simulink model "mct_ut"  (Simulink 8.1)
settings: Solver=FixedStepDiscrete  StartTime=0.0  StopTime=Inf  FixedStep=0.005  RelTol=1e-3
libraries: siltestlib x41, mct x1
settings Model: Creator=xsellart  LastModifiedBy=AT015555
settings DataIOCC: SignalLoggingSaveFormat=Dataset
settings OptimizationCC: ExpressionDepthLimit=128
settings DebuggingCC: FcnCallInpInsideContextMsg=EnableAllAsError
settings GRTTargetCC: CombineOutputUpdateFcns=on  GRTInterface=off

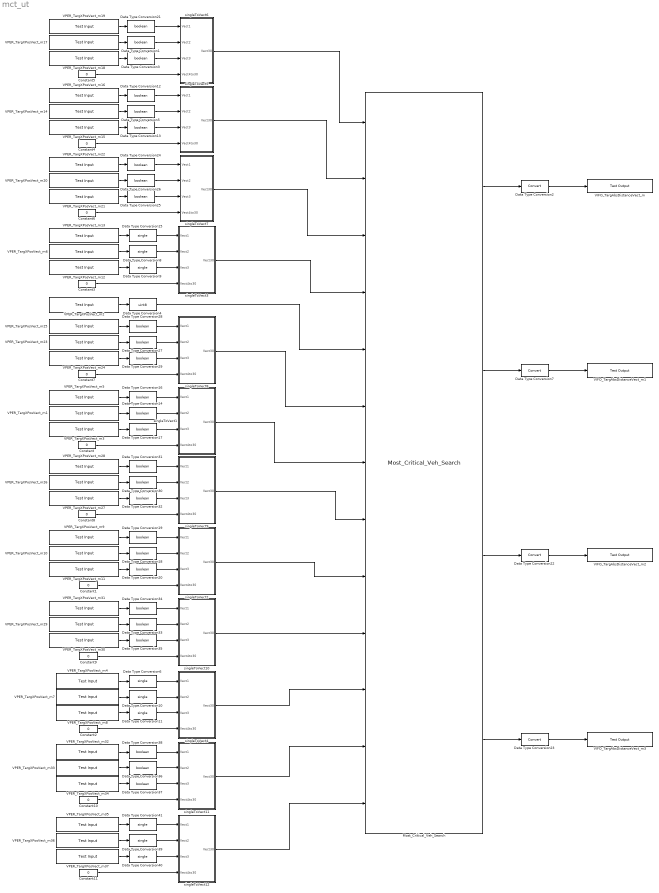
== system mct_ut ==
  Constant{,1,4..10} (9 alike) : Constant  Value=0  OutDataTypeStr=boolean
  Constant11 : Constant  Value=0  OutDataTypeStr=single
  Constant2 : Constant  Value=0  OutDataTypeStr=single
  Constant3 : Constant  Value=0  OutDataTypeStr=single
  Data Type Conversion{1,3,5,12..14,16..21,24..38} (27 alike) : DataTypeConversion  OutDataTypeStr=boolean
  Data Type Conversion{6,8..11,15,39..41} (9 alike) : DataTypeConversion  OutDataTypeStr=single
  Data Type Conversion{2,7,22..23} (4 alike) : DataTypeConversion
  Data Type Conversion4 : DataTypeConversion  OutDataTypeStr=uint8
  Most_Critical_Veh_Search : mct/Most_Critical_Veh_Search
  VIFO_TargAbsDistanceVect_m : siltestlib/Test Output  varname=VIFO_FCWMCTTargId_num  sampletime=-1
  VIFO_TargAbsDistanceVect_m1 : siltestlib/Test Output  varname=VIFO_AEBMCTTargId_num  sampletime=-1
  VIFO_TargAbsDistanceVect_m2 : siltestlib/Test Output  varname=VIFO_ACCMCTTargId_num  sampletime=-1
  VIFO_TargAbsDistanceVect_m3 : siltestlib/Test Output  varname=VIFO_VRUMCTTargId_num  sampletime=-1
  VPER_TargXPosVect_m1 : siltestlib/Test Input  varname=VIFO_ACCTargetIsVehVect30_flg2  sampletime=0.005
  VPER_TargXPosVect_m10 : siltestlib/Test Input  varname=VIFO_AEBTargetSameDirVect30_flg2  sampletime=0.005
  VPER_TargXPosVect_m11 : siltestlib/Test Input  varname=VIFO_AEBTargetSameDirVect30_flg3  sampletime=0.005
  VPER_TargXPosVect_m12 : siltestlib/Test Input  varname=VIFO_TargAbsDistanceVect30_m3  sampletime=0.005
  VPER_TargXPosVect_m13 : siltestlib/Test Input  varname=VIFO_TargAbsDistanceVect30_m1  sampletime=0.005
  VPER_TargXPosVect_m14 : siltestlib/Test Input  varname=VIFO_AEBVehInPathVect30_flg2  sampletime=0.005
  VPER_TargXPosVect_m15 : siltestlib/Test Input  varname=VIFO_AEBVehInPathVect30_flg3  sampletime=0.005
  VPER_TargXPosVect_m16 : siltestlib/Test Input  varname=VIFO_AEBVehInPathVect30_flg1  sampletime=0.005
  VPER_TargXPosVect_m17 : siltestlib/Test Input  varname=VIFO_FCWVehInPathVect30_flg2  sampletime=0.005
  VPER_TargXPosVect_m18 : siltestlib/Test Input  varname=VIFO_FCWVehInPathVect30_flg3  sampletime=0.005
  VPER_TargXPosVect_m19 : siltestlib/Test Input  varname=VIFO_FCWVehInPathVect30_flg1  sampletime=0.005
  VPER_TargXPosVect_m2 : siltestlib/Test Input  varname=VPER_NumberOfTargets_enum  sampletime=0.005
  VPER_TargXPosVect_m20 : siltestlib/Test Input  varname=VIFO_ACCVehInPathVect30_flg2  sampletime=0.005
  VPER_TargXPosVect_m21 : siltestlib/Test Input  varname=VIFO_ACCVehInPathVect30_flg3  sampletime=0.005
  VPER_TargXPosVect_m22 : siltestlib/Test Input  varname=VIFO_ACCVehInPathVect30_flg1  sampletime=0.005
  VPER_TargXPosVect_m23 : siltestlib/Test Input  varname=VIFO_AEBTargetIsVehVect30_flg2  sampletime=0.005
  VPER_TargXPosVect_m24 : siltestlib/Test Input  varname=VIFO_AEBTargetIsVehVect30_flg3  sampletime=0.005
  VPER_TargXPosVect_m25 : siltestlib/Test Input  varname=VIFO_AEBTargetIsVehVect30_flg1  sampletime=0.005
  VPER_TargXPosVect_m26 : siltestlib/Test Input  varname=VIFO_VRUTargetIsPedVect30_flg2  sampletime=0.005
  VPER_TargXPosVect_m27 : siltestlib/Test Input  varname=VIFO_VRUTargetIsPedVect30_flg3  sampletime=0.005
  VPER_TargXPosVect_m28 : siltestlib/Test Input  varname=VIFO_VRUTargetIsPedVect30_flg1  sampletime=0.005
  VPER_TargXPosVect_m29 : siltestlib/Test Input  varname=VIFO_ACCTargetSameDirVect30_flg2  sampletime=0.005
  VPER_TargXPosVect_m3 : siltestlib/Test Input  varname=VIFO_ACCTargetIsVehVect30_flg3  sampletime=0.005
  VPER_TargXPosVect_m30 : siltestlib/Test Input  varname=VIFO_ACCTargetSameDirVect30_flg3  sampletime=0.005
  VPER_TargXPosVect_m31 : siltestlib/Test Input  varname=VIFO_ACCTargetSameDirVect30_flg1  sampletime=0.005
  VPER_TargXPosVect_m32 : siltestlib/Test Input  varname=VIFO_VRUIsPotentialVect30_flg1  sampletime=0.005
  VPER_TargXPosVect_m33 : siltestlib/Test Input  varname=VIFO_VRUIsPotentialVect30_flg2  sampletime=0.005
  VPER_TargXPosVect_m34 : siltestlib/Test Input  varname=VIFO_VRUIsPotentialVect30_flg3  sampletime=0.005
  VPER_TargXPosVect_m35 : siltestlib/Test Input  varname=VIFO_VRUSingleTTCVect30_s1  sampletime=0.005
  VPER_TargXPosVect_m36 : siltestlib/Test Input  varname=VIFO_VRUSingleTTCVect30_s2  sampletime=0.005
  VPER_TargXPosVect_m37 : siltestlib/Test Input  varname=VIFO_VRUSingleTTCVect30_s3  sampletime=0.005
  VPER_TargXPosVect_m4 : siltestlib/Test Input  varname=VPER_TargExisProbVect30_num1  sampletime=0.005
  VPER_TargXPosVect_m5 : siltestlib/Test Input  varname=VIFO_ACCTargetIsVehVect30_flg1  sampletime=0.005
  VPER_TargXPosVect_m6 : siltestlib/Test Input  varname=VIFO_TargAbsDistanceVect30_m2  sampletime=0.005
  VPER_TargXPosVect_m7 : siltestlib/Test Input  varname=VPER_TargExisProbVect30_num2  sampletime=0.005
  VPER_TargXPosVect_m8 : siltestlib/Test Input  varname=VPER_TargExisProbVect30_num3  sampletime=0.005
  VPER_TargXPosVect_m9 : siltestlib/Test Input  varname=VIFO_AEBTargetSameDirVect30_flg1  sampletime=0.005
  singleToVect1 : Subsystem
  singleToVect10 : Subsystem
  singleToVect11 : Subsystem
  singleToVect12 : Subsystem
  singleToVect2 : Subsystem
  singleToVect3 : Subsystem
  singleToVect4 : Subsystem
  singleToVect5 : Subsystem
  singleToVect6 : Subsystem
  singleToVect7 : Subsystem
  singleToVect8 : Subsystem
  singleToVect9 : Subsystem
  wires:
  Most_Critical_Veh_Search/1 -> Data Type Conversion2/1
  Data Type Conversion2/1 -> VIFO_TargAbsDistanceVect_m/1
  VPER_TargXPosVect_m2/1 -> Data Type Conversion4/1
  VPER_TargXPosVect_m4/1 -> Data Type Conversion6/1
  Data Type Conversion6/1 -> singleToVect4/1(Vect1)
  Most_Critical_Veh_Search/2 -> Data Type Conversion7/1
  Data Type Conversion7/1 -> VIFO_TargAbsDistanceVect_m1/1
  VPER_TargXPosVect_m7/1 -> Data Type Conversion10/1
  Data Type Conversion10/1 -> singleToVect4/2(Vect2)
  VPER_TargXPosVect_m8/1 -> Data Type Conversion11/1
  Data Type Conversion11/1 -> singleToVect4/3(Vect3)
  VPER_TargXPosVect_m9/1 -> Data Type Conversion19/1
  Data Type Conversion19/1 -> singleToVect2/1(Vect1)
  VPER_TargXPosVect_m10/1 -> Data Type Conversion18/1
  Data Type Conversion18/1 -> singleToVect2/2(Vect2)
  VPER_TargXPosVect_m11/1 -> Data Type Conversion20/1
  Data Type Conversion20/1 -> singleToVect2/3(Vect3)
  VPER_TargXPosVect_m5/1 -> Data Type Conversion16/1
  Data Type Conversion16/1 -> singleToVect1/1(Vect1)
  VPER_TargXPosVect_m1/1 -> Data Type Conversion14/1
  Data Type Conversion14/1 -> singleToVect1/2(Vect2)
  VPER_TargXPosVect_m3/1 -> Data Type Conversion17/1
  Data Type Conversion17/1 -> singleToVect1/3(Vect3)
  VPER_TargXPosVect_m13/1 -> Data Type Conversion15/1
  Data Type Conversion15/1 -> singleToVect3/1(Vect1)
  VPER_TargXPosVect_m6/1 -> Data Type Conversion8/1
  Data Type Conversion8/1 -> singleToVect3/2(Vect2)
  VPER_TargXPosVect_m12/1 -> Data Type Conversion9/1
  Data Type Conversion9/1 -> singleToVect3/3(Vect3)
  VPER_TargXPosVect_m16/1 -> Data Type Conversion12/1
  Data Type Conversion12/1 -> singleToVect5/1(Vect1)
  VPER_TargXPosVect_m14/1 -> Data Type Conversion5/1
  Data Type Conversion5/1 -> singleToVect5/2(Vect2)
  VPER_TargXPosVect_m15/1 -> Data Type Conversion13/1
  Data Type Conversion13/1 -> singleToVect5/3(Vect3)
  singleToVect5/1(Vect30) -> Most_Critical_Veh_Search/2
  VPER_TargXPosVect_m19/1 -> Data Type Conversion21/1
  Data Type Conversion21/1 -> singleToVect6/1(Vect1)
  VPER_TargXPosVect_m17/1 -> Data Type Conversion1/1
  Data Type Conversion1/1 -> singleToVect6/2(Vect2)
  VPER_TargXPosVect_m18/1 -> Data Type Conversion3/1
  Data Type Conversion3/1 -> singleToVect6/3(Vect3)
  singleToVect6/1(Vect30) -> Most_Critical_Veh_Search/1
  Constant/1 -> singleToVect1/4(Vect4to30)
  Constant1/1 -> singleToVect2/4(Vect4to30)
  Constant2/1 -> singleToVect4/4(Vect4to30)
  Constant3/1 -> singleToVect3/4(Vect4to30)
  Constant4/1 -> singleToVect5/4(Vect4to30)
  Constant5/1 -> singleToVect6/4(Vect4to30)
  Data Type Conversion22/1 -> VIFO_TargAbsDistanceVect_m2/1
  Data Type Conversion23/1 -> VIFO_TargAbsDistanceVect_m3/1
  Most_Critical_Veh_Search/3 -> Data Type Conversion22/1
  Most_Critical_Veh_Search/4 -> Data Type Conversion23/1
  VPER_TargXPosVect_m22/1 -> Data Type Conversion24/1
  Data Type Conversion24/1 -> singleToVect7/1(Vect1)
  VPER_TargXPosVect_m20/1 -> Data Type Conversion26/1
  Data Type Conversion26/1 -> singleToVect7/2(Vect2)
  VPER_TargXPosVect_m21/1 -> Data Type Conversion25/1
  Data Type Conversion25/1 -> singleToVect7/3(Vect3)
  Constant6/1 -> singleToVect7/4(Vect4to30)
  singleToVect7/1(Vect30) -> Most_Critical_Veh_Search/3
  singleToVect3/1(Vect30) -> Most_Critical_Veh_Search/4
  Data Type Conversion4/1 -> Most_Critical_Veh_Search/5
  VPER_TargXPosVect_m25/1 -> Data Type Conversion28/1
  Data Type Conversion28/1 -> singleToVect8/1(Vect1)
  VPER_TargXPosVect_m23/1 -> Data Type Conversion27/1
  Data Type Conversion27/1 -> singleToVect8/2(Vect2)
  VPER_TargXPosVect_m24/1 -> Data Type Conversion29/1
  Data Type Conversion29/1 -> singleToVect8/3(Vect3)
  Constant7/1 -> singleToVect8/4(Vect4to30)
  singleToVect8/1(Vect30) -> Most_Critical_Veh_Search/6
  singleToVect1/1(Vect30) -> Most_Critical_Veh_Search/7
  VPER_TargXPosVect_m28/1 -> Data Type Conversion31/1
  Data Type Conversion31/1 -> singleToVect9/1(Vect1)
  VPER_TargXPosVect_m26/1 -> Data Type Conversion30/1
  Data Type Conversion30/1 -> singleToVect9/2(Vect2)
  VPER_TargXPosVect_m27/1 -> Data Type Conversion32/1
  Data Type Conversion32/1 -> singleToVect9/3(Vect3)
  Constant8/1 -> singleToVect9/4(Vect4to30)
  singleToVect9/1(Vect30) -> Most_Critical_Veh_Search/8
  singleToVect2/1(Vect30) -> Most_Critical_Veh_Search/9
  VPER_TargXPosVect_m31/1 -> Data Type Conversion34/1
  Data Type Conversion34/1 -> singleToVect10/1(Vect1)
  VPER_TargXPosVect_m29/1 -> Data Type Conversion33/1
  Data Type Conversion33/1 -> singleToVect10/2(Vect2)
  VPER_TargXPosVect_m30/1 -> Data Type Conversion35/1
  Data Type Conversion35/1 -> singleToVect10/3(Vect3)
  Constant9/1 -> singleToVect10/4(Vect4to30)
  singleToVect10/1(Vect30) -> Most_Critical_Veh_Search/10
  VPER_TargXPosVect_m32/1 -> Data Type Conversion38/1
  Data Type Conversion38/1 -> singleToVect11/1(Vect1)
  VPER_TargXPosVect_m33/1 -> Data Type Conversion36/1
  Data Type Conversion36/1 -> singleToVect11/2(Vect2)
  VPER_TargXPosVect_m34/1 -> Data Type Conversion37/1
  Data Type Conversion37/1 -> singleToVect11/3(Vect3)
  Constant10/1 -> singleToVect11/4(Vect4to30)
  VPER_TargXPosVect_m35/1 -> Data Type Conversion41/1
  Data Type Conversion41/1 -> singleToVect12/1(Vect1)
  VPER_TargXPosVect_m36/1 -> Data Type Conversion39/1
  Data Type Conversion39/1 -> singleToVect12/2(Vect2)
  VPER_TargXPosVect_m37/1 -> Data Type Conversion40/1
  Data Type Conversion40/1 -> singleToVect12/3(Vect3)
  Constant11/1 -> singleToVect12/4(Vect4to30)
  singleToVect12/1(Vect30) -> Most_Critical_Veh_Search/13
  singleToVect4/1(Vect30) -> Most_Critical_Veh_Search/11
  singleToVect11/1(Vect30) -> Most_Critical_Veh_Search/12

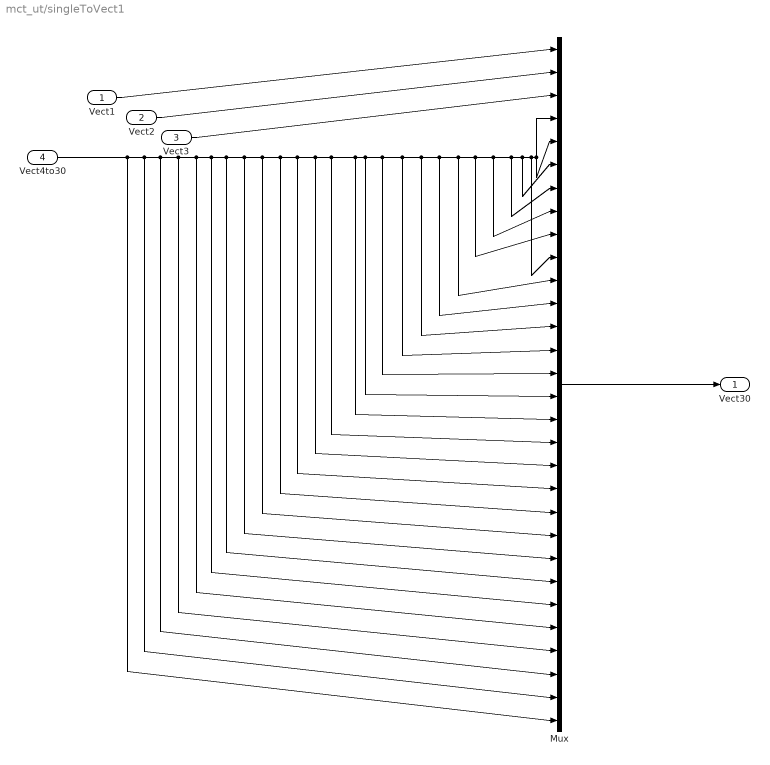
== system mct_ut/singleToVect1 ==
  Vect1 : Inport
  Vect2 : Inport  Port=2
  Vect3 : Inport  Port=3
  Vect4to30 : Inport  Port=4
  Mux : Mux  Inputs=30
  Vect30 : Outport
  wires:
  Mux/1 -> Vect30/1
  Vect4to30/1 -> Mux/30, Mux/29, Mux/28, Mux/27, Mux/26, Mux/25, Mux/24, Mux/23, Mux/22, Mux/21, Mux/20, Mux/19, Mux/18, Mux/17, Mux/16, Mux/15, Mux/14, Mux/13, Mux/12, Mux/11, Mux/10, Mux/4, Mux/5, Mux/6, Mux/7, Mux/8, Mux/9
  Vect3/1 -> Mux/3
  Vect2/1 -> Mux/2
  Vect1/1 -> Mux/1

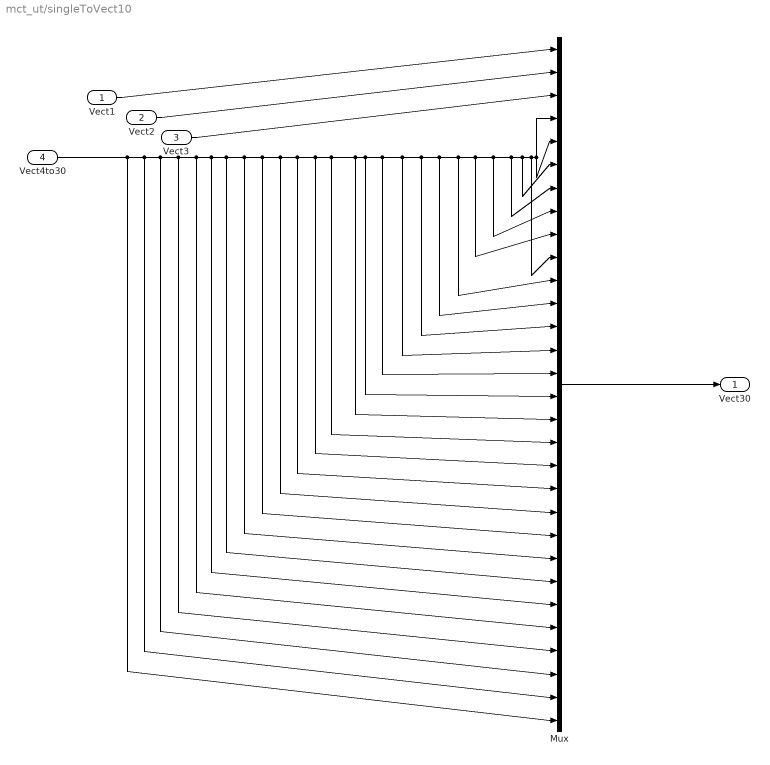
== system mct_ut/singleToVect10 ==
  Vect1 : Inport
  Vect2 : Inport  Port=2
  Vect3 : Inport  Port=3
  Vect4to30 : Inport  Port=4
  Mux : Mux  Inputs=30
  Vect30 : Outport
  wires:
  Vect1/1 -> Mux/1
  Vect2/1 -> Mux/2
  Vect3/1 -> Mux/3
  Vect4to30/1 -> Mux/9, Mux/8, Mux/7, Mux/6, Mux/5, Mux/4, Mux/10, Mux/11, Mux/12, Mux/13, Mux/14, Mux/15, Mux/16, Mux/17, Mux/18, Mux/19, Mux/20, Mux/21, Mux/22, Mux/23, Mux/24, Mux/25, Mux/26, Mux/27, Mux/28, Mux/29, Mux/30
  Mux/1 -> Vect30/1

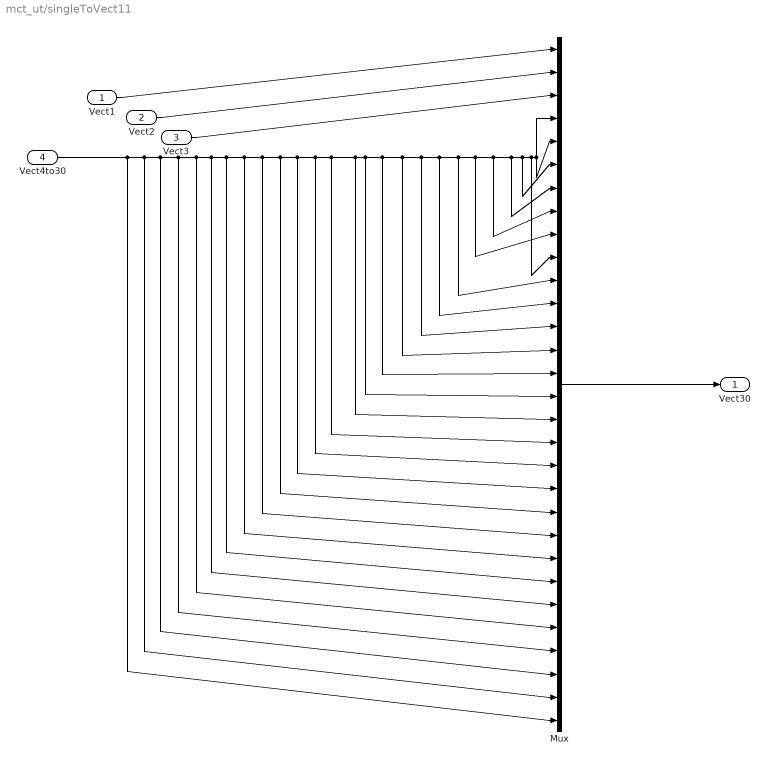
== system mct_ut/singleToVect11 ==
  Vect1 : Inport
  Vect2 : Inport  Port=2
  Vect3 : Inport  Port=3
  Vect4to30 : Inport  Port=4
  Mux : Mux  Inputs=30
  Vect30 : Outport
  wires:
  Vect1/1 -> Mux/1
  Vect2/1 -> Mux/2
  Vect3/1 -> Mux/3
  Vect4to30/1 -> Mux/9, Mux/8, Mux/7, Mux/6, Mux/5, Mux/4, Mux/10, Mux/11, Mux/12, Mux/13, Mux/14, Mux/15, Mux/16, Mux/17, Mux/18, Mux/19, Mux/20, Mux/21, Mux/22, Mux/23, Mux/24, Mux/25, Mux/26, Mux/27, Mux/28, Mux/29, Mux/30
  Mux/1 -> Vect30/1

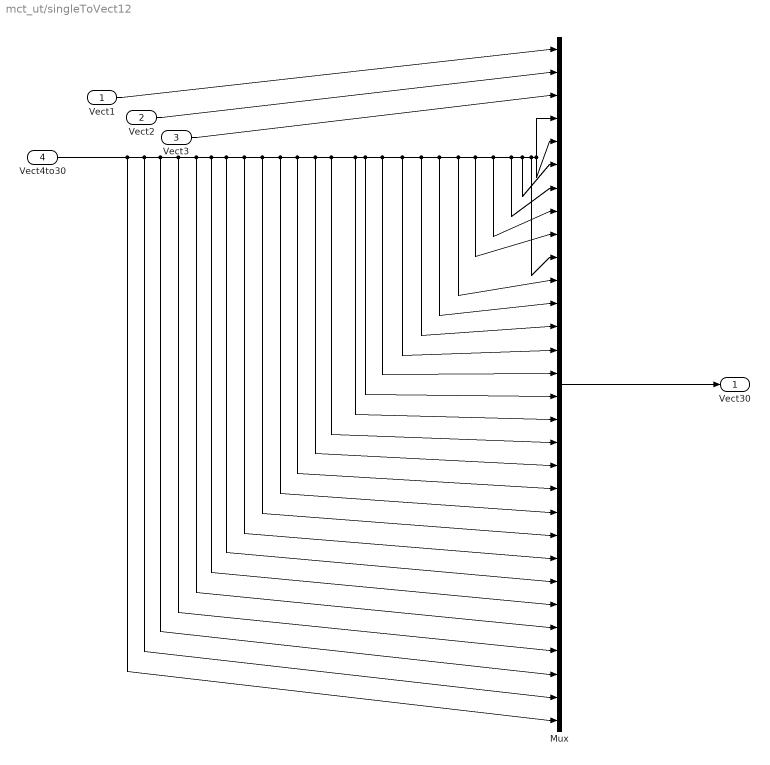
== system mct_ut/singleToVect12 ==
  Vect1 : Inport
  Vect2 : Inport  Port=2
  Vect3 : Inport  Port=3
  Vect4to30 : Inport  Port=4
  Mux : Mux  Inputs=30
  Vect30 : Outport
  wires:
  Mux/1 -> Vect30/1
  Vect4to30/1 -> Mux/30, Mux/29, Mux/28, Mux/27, Mux/26, Mux/25, Mux/24, Mux/23, Mux/22, Mux/21, Mux/20, Mux/19, Mux/18, Mux/17, Mux/16, Mux/15, Mux/14, Mux/13, Mux/12, Mux/11, Mux/10, Mux/4, Mux/5, Mux/6, Mux/7, Mux/8, Mux/9
  Vect3/1 -> Mux/3
  Vect2/1 -> Mux/2
  Vect1/1 -> Mux/1

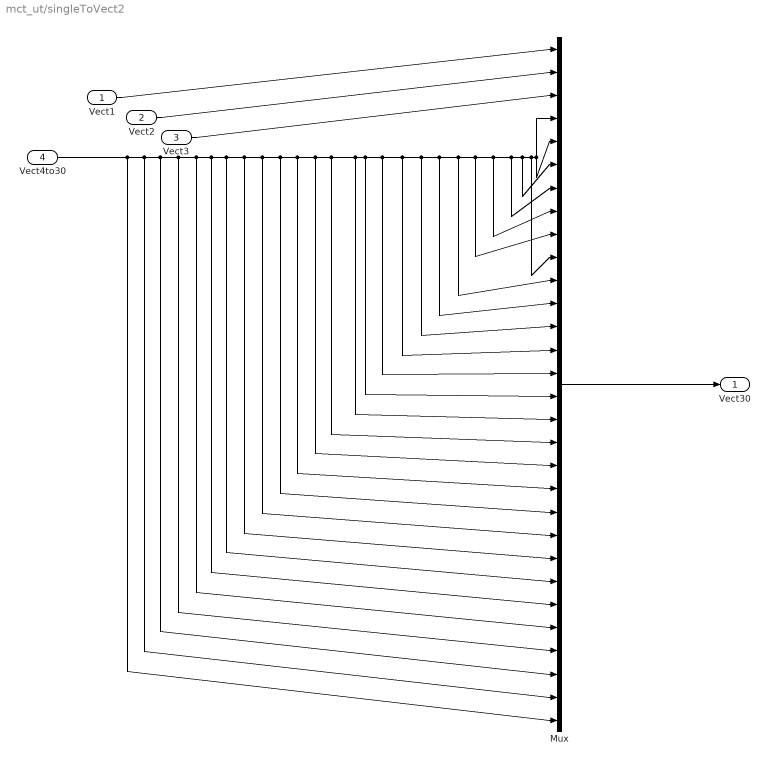
== system mct_ut/singleToVect2 ==
  Vect1 : Inport
  Vect2 : Inport  Port=2
  Vect3 : Inport  Port=3
  Vect4to30 : Inport  Port=4
  Mux : Mux  Inputs=30
  Vect30 : Outport
  wires:
  Mux/1 -> Vect30/1
  Vect4to30/1 -> Mux/30, Mux/29, Mux/28, Mux/27, Mux/26, Mux/25, Mux/24, Mux/23, Mux/22, Mux/21, Mux/20, Mux/19, Mux/18, Mux/17, Mux/16, Mux/15, Mux/14, Mux/13, Mux/12, Mux/11, Mux/10, Mux/4, Mux/5, Mux/6, Mux/7, Mux/8, Mux/9
  Vect3/1 -> Mux/3
  Vect2/1 -> Mux/2
  Vect1/1 -> Mux/1

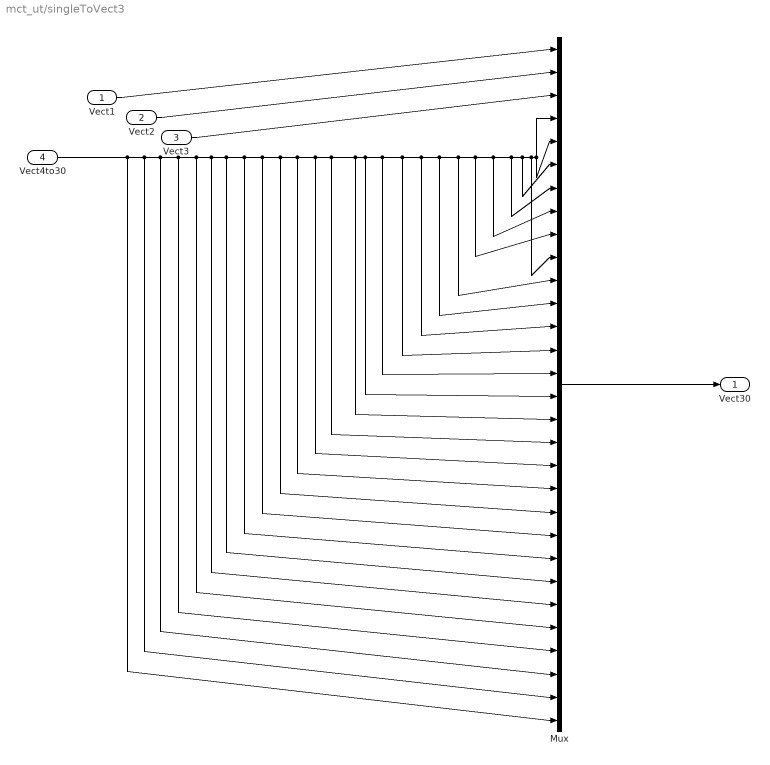
== system mct_ut/singleToVect3 ==
  Vect1 : Inport
  Vect2 : Inport  Port=2
  Vect3 : Inport  Port=3
  Vect4to30 : Inport  Port=4
  Mux : Mux  Inputs=30
  Vect30 : Outport
  wires:
  Mux/1 -> Vect30/1
  Vect4to30/1 -> Mux/30, Mux/29, Mux/28, Mux/27, Mux/26, Mux/25, Mux/24, Mux/23, Mux/22, Mux/21, Mux/20, Mux/19, Mux/18, Mux/17, Mux/16, Mux/15, Mux/14, Mux/13, Mux/12, Mux/11, Mux/10, Mux/4, Mux/5, Mux/6, Mux/7, Mux/8, Mux/9
  Vect3/1 -> Mux/3
  Vect2/1 -> Mux/2
  Vect1/1 -> Mux/1

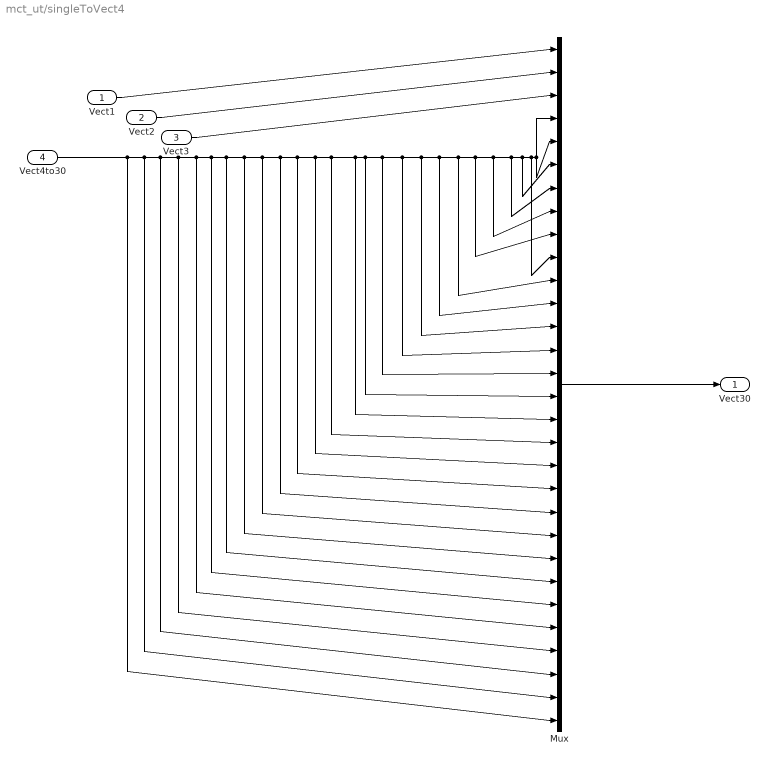
== system mct_ut/singleToVect4 ==
  Vect1 : Inport
  Vect2 : Inport  Port=2
  Vect3 : Inport  Port=3
  Vect4to30 : Inport  Port=4
  Mux : Mux  Inputs=30
  Vect30 : Outport
  wires:
  Mux/1 -> Vect30/1
  Vect4to30/1 -> Mux/30, Mux/29, Mux/28, Mux/27, Mux/26, Mux/25, Mux/24, Mux/23, Mux/22, Mux/21, Mux/20, Mux/19, Mux/18, Mux/17, Mux/16, Mux/15, Mux/14, Mux/13, Mux/12, Mux/11, Mux/10, Mux/4, Mux/5, Mux/6, Mux/7, Mux/8, Mux/9
  Vect3/1 -> Mux/3
  Vect2/1 -> Mux/2
  Vect1/1 -> Mux/1

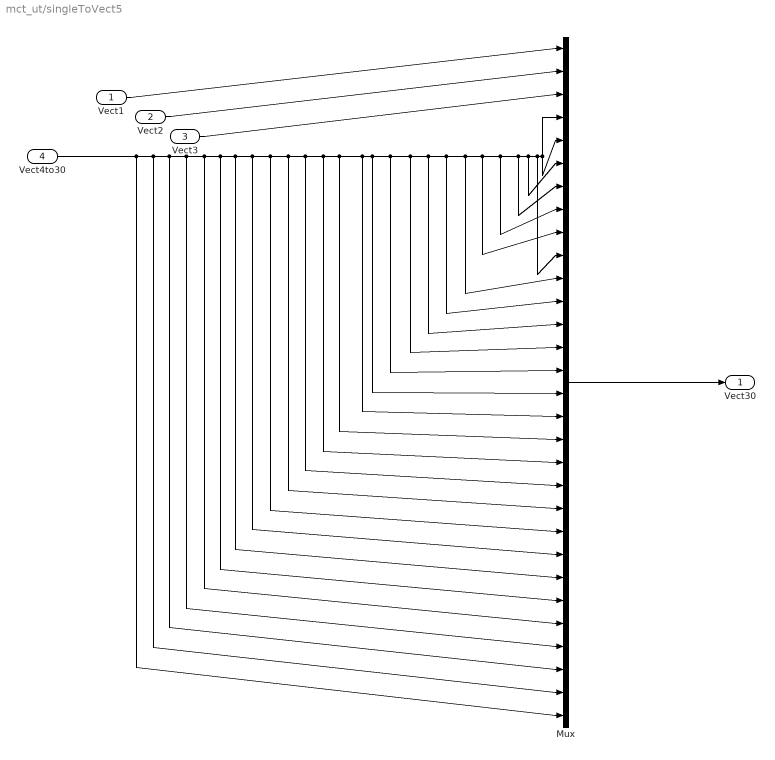
== system mct_ut/singleToVect5 ==
  Vect1 : Inport
  Vect2 : Inport  Port=2
  Vect3 : Inport  Port=3
  Vect4to30 : Inport  Port=4
  Mux : Mux  Inputs=30
  Vect30 : Outport
  wires:
  Mux/1 -> Vect30/1
  Vect4to30/1 -> Mux/30, Mux/29, Mux/28, Mux/27, Mux/26, Mux/25, Mux/24, Mux/23, Mux/22, Mux/21, Mux/20, Mux/19, Mux/18, Mux/17, Mux/16, Mux/15, Mux/14, Mux/13, Mux/12, Mux/11, Mux/10, Mux/4, Mux/5, Mux/6, Mux/7, Mux/8, Mux/9
  Vect3/1 -> Mux/3
  Vect2/1 -> Mux/2
  Vect1/1 -> Mux/1

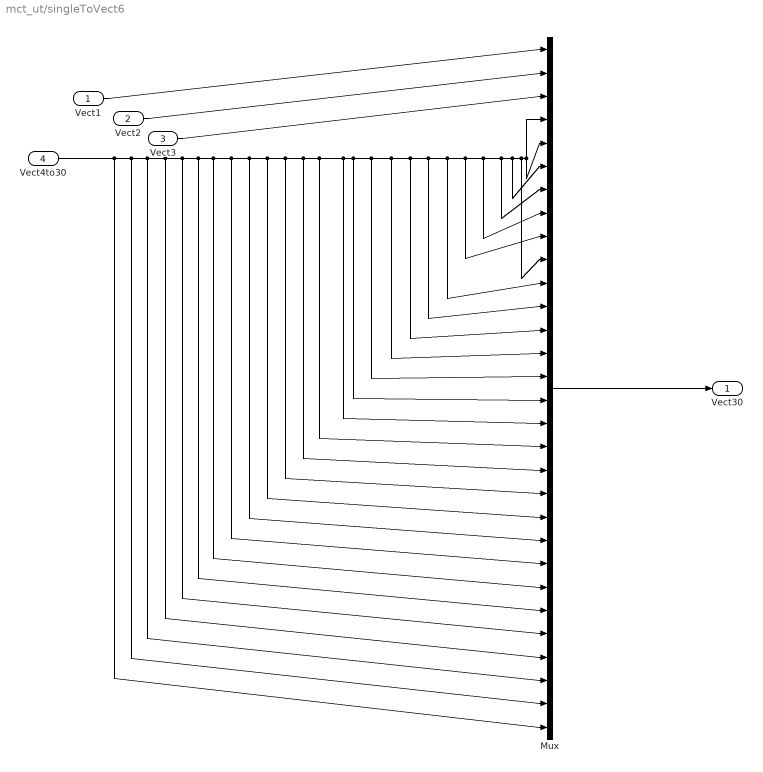
== system mct_ut/singleToVect6 ==
  Vect1 : Inport
  Vect2 : Inport  Port=2
  Vect3 : Inport  Port=3
  Vect4to30 : Inport  Port=4
  Mux : Mux  Inputs=30
  Vect30 : Outport
  wires:
  Mux/1 -> Vect30/1
  Vect4to30/1 -> Mux/30, Mux/29, Mux/28, Mux/27, Mux/26, Mux/25, Mux/24, Mux/23, Mux/22, Mux/21, Mux/20, Mux/19, Mux/18, Mux/17, Mux/16, Mux/15, Mux/14, Mux/13, Mux/12, Mux/11, Mux/10, Mux/4, Mux/5, Mux/6, Mux/7, Mux/8, Mux/9
  Vect3/1 -> Mux/3
  Vect2/1 -> Mux/2
  Vect1/1 -> Mux/1

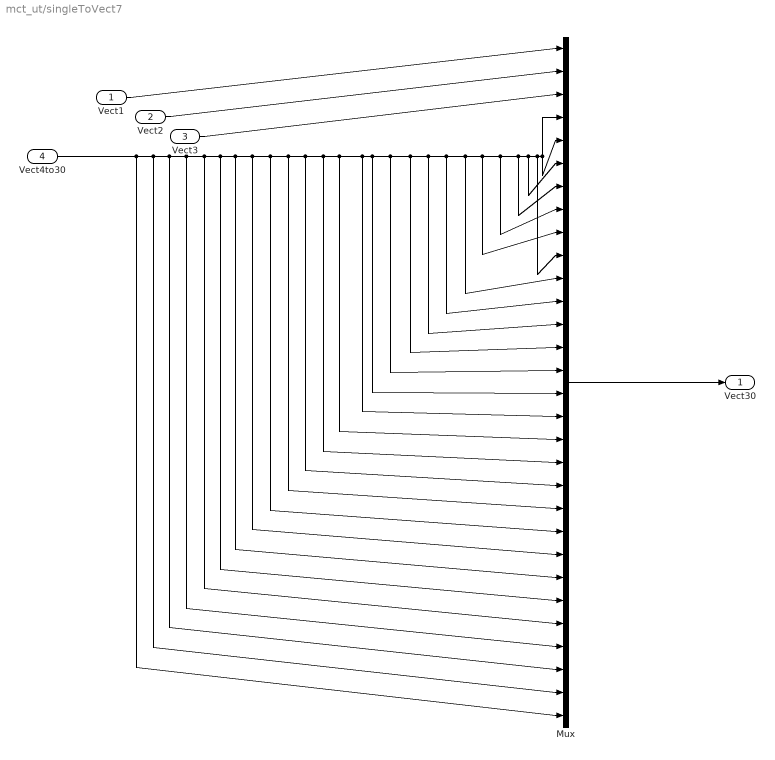
== system mct_ut/singleToVect7 ==
  Vect1 : Inport
  Vect2 : Inport  Port=2
  Vect3 : Inport  Port=3
  Vect4to30 : Inport  Port=4
  Mux : Mux  Inputs=30
  Vect30 : Outport
  wires:
  Vect1/1 -> Mux/1
  Vect2/1 -> Mux/2
  Vect3/1 -> Mux/3
  Vect4to30/1 -> Mux/9, Mux/8, Mux/7, Mux/6, Mux/5, Mux/4, Mux/10, Mux/11, Mux/12, Mux/13, Mux/14, Mux/15, Mux/16, Mux/17, Mux/18, Mux/19, Mux/20, Mux/21, Mux/22, Mux/23, Mux/24, Mux/25, Mux/26, Mux/27, Mux/28, Mux/29, Mux/30
  Mux/1 -> Vect30/1

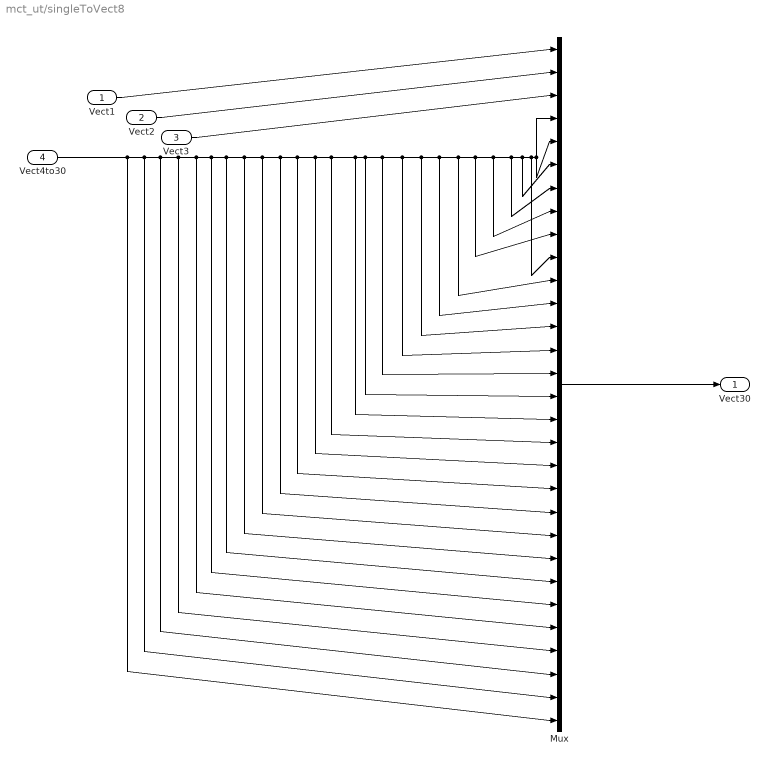
== system mct_ut/singleToVect8 ==
  Vect1 : Inport
  Vect2 : Inport  Port=2
  Vect3 : Inport  Port=3
  Vect4to30 : Inport  Port=4
  Mux : Mux  Inputs=30
  Vect30 : Outport
  wires:
  Vect1/1 -> Mux/1
  Vect2/1 -> Mux/2
  Vect3/1 -> Mux/3
  Vect4to30/1 -> Mux/9, Mux/8, Mux/7, Mux/6, Mux/5, Mux/4, Mux/10, Mux/11, Mux/12, Mux/13, Mux/14, Mux/15, Mux/16, Mux/17, Mux/18, Mux/19, Mux/20, Mux/21, Mux/22, Mux/23, Mux/24, Mux/25, Mux/26, Mux/27, Mux/28, Mux/29, Mux/30
  Mux/1 -> Vect30/1

== system mct_ut/singleToVect9 ==
  Vect1 : Inport
  Vect2 : Inport  Port=2
  Vect3 : Inport  Port=3
  Vect4to30 : Inport  Port=4
  Mux : Mux  Inputs=30
  Vect30 : Outport
  wires:
  Vect1/1 -> Mux/1
  Vect2/1 -> Mux/2
  Vect3/1 -> Mux/3
  Vect4to30/1 -> Mux/9, Mux/8, Mux/7, Mux/6, Mux/5, Mux/4, Mux/10, Mux/11, Mux/12, Mux/13, Mux/14, Mux/15, Mux/16, Mux/17, Mux/18, Mux/19, Mux/20, Mux/21, Mux/22, Mux/23, Mux/24, Mux/25, Mux/26, Mux/27, Mux/28, Mux/29, Mux/30
  Mux/1 -> Vect30/1
